simulink model "sampleModel161"  (R2021b)
settings: Solver=VariableStepAuto  StartTime=0.0  StopTime=10.0  RelTol=1e-3
undefined symbols (not defined in the file or in its folder): DiscIntNeverNeededParam
libraries: simulink x19, slpidlib x1
settings Model: Creator=user  LastModifiedBy=user

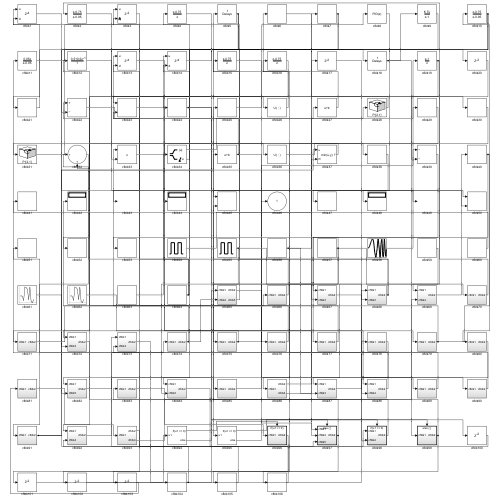
[thumbnail: Simulink's stored preview of the top-level diagram]
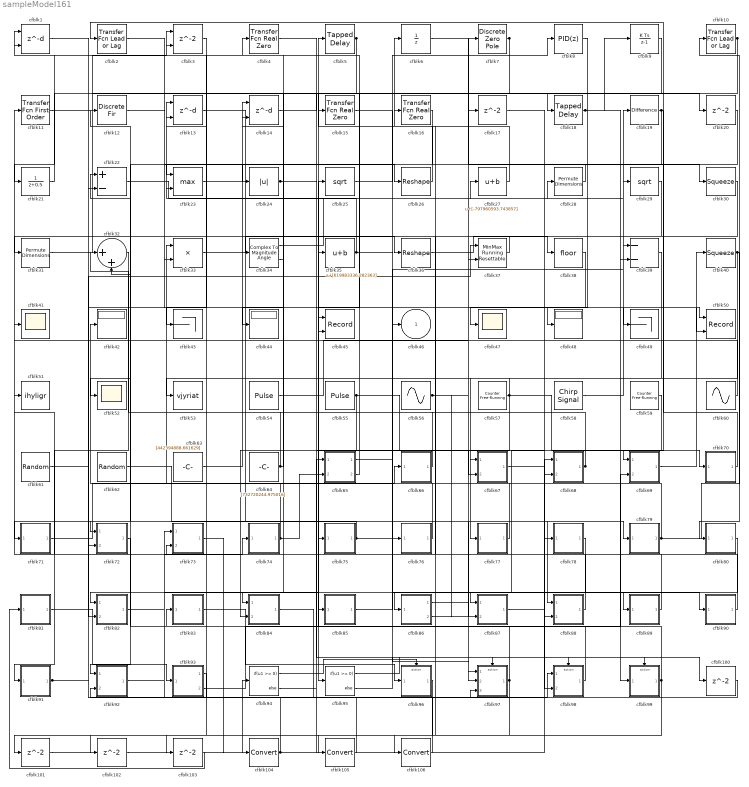
== system sampleModel161 ==
  cfblk1 : Delay  DelayLengthSource=Input port  SampleTime=1
      settings: InputPortMap=u0,p1
  cfblk10 : simulink/Discrete/Transfer Fcn Lead or Lag  PoleZ=0.95  ZeroZ=0.75  ICPrevOutput=0.0  ICPrevInput=0.0  DoSatur=off
      settings: SourceProductBaseCode=SL
  cfblk{17,20,100..103} (6 alike) : Delay  SampleTime=1
  cfblk104 : DataTypeConversion
  cfblk105 : DataTypeConversion
  cfblk106 : DataTypeConversion
  cfblk11 : simulink/Discrete/Transfer Fcn First Order  PoleZ=0.95  ICPrevOutput=0.0  DoSatur=off
  cfblk12 : DiscreteFir  SampleTime=1
  cfblk13 : Delay  DelayLengthSource=Input port  SampleTime=1
      settings: InputPortMap=u0,p1
  cfblk14 : Delay  DelayLengthSource=Input port  SampleTime=1
      settings: InputPortMap=u0,p1
  cfblk15 : simulink/Discrete/Transfer Fcn Real Zero  ZeroZ=0.75  ICPrevInput=0.0  DoSatur=off
      settings: SourceProductBaseCode=SL
  cfblk16 : simulink/Discrete/Transfer Fcn Real Zero  ZeroZ=0.75  ICPrevInput=0.0  DoSatur=off
      settings: SourceProductBaseCode=SL
  cfblk18 : simulink/Discrete/Tapped Delay  vinit=0.0  samptime=-1  NumDelays=1  DelayOrder=Oldest  includeCurrent=off
  cfblk19 : simulink/Discrete/Difference  ICPrevInput=0.0  OutMin=[]  OutMax=[]  OutDataTypeStr=Inherit: Inherit via back propagation  OutDataType=fixdt(1, 16)  OutScaling=2^-10  DoSatur=off
  cfblk2 : simulink/Discrete/Transfer Fcn Lead or Lag  PoleZ=0.95  ZeroZ=0.75  ICPrevOutput=0.0  ICPrevInput=0.0  DoSatur=off
      settings: SourceProductBaseCode=SL
  cfblk21 : DiscreteTransferFcn  SampleTime=1
  cfblk22 : Sum  Inputs=+-
  cfblk23 : MinMax  Function=max  Inputs=2
  cfblk24 : Abs
  cfblk25 : Sqrt  SaturateOnIntegerOverflow=on
  cfblk26 : Reshape
  cfblk27 : Bias  Bias=[-797960593.743857]
  cfblk28 : PermuteDimensions
  cfblk29 : Sqrt  SaturateOnIntegerOverflow=on
  cfblk3 : Delay  ShowEnablePort=on  SampleTime=1
      settings: InputPortMap=u0,e6
  cfblk30 : Squeeze
  cfblk31 : PermuteDimensions
  cfblk32 : Sum  Inputs=|++
  cfblk33 : Product  Inputs=**
  cfblk34 : ComplexToMagnitudeAngle
  cfblk35 : Bias  Bias=[619983336.282363]
  cfblk36 : Reshape
  cfblk37 : simulink/Math Operations/MinMax Running Resettable  Function=min  vinit=0.0
  cfblk38 : Rounding
  cfblk39 : Sum  Inputs=--
  cfblk4 : simulink/Discrete/Transfer Fcn Real Zero  ZeroZ=0.75  ICPrevInput=0.0  DoSatur=off
      settings: SourceProductBaseCode=SL
  cfblk40 : Squeeze
  cfblk41 : Scope
  cfblk42 : Display
  cfblk43 : Terminator
  cfblk44 : Display
  cfblk45 : Record  FileSettingsInternal="{\"entries\":[{\"content\":{\"excelSettings\":{\"content\":{},\"type\":\"Streamout.ExcelSettings\"}},\"type\":\"Streamout.FileSettingStorage\",\"uuid\":\"aea9327c-655b-48bd-a78c-8c98bb394b7e\"}],\"packageUris\":[\"http://schema.mathworks.com/mf0/streamout_blocks/R2020a\"],\"version\":\"1.0\"}"  Layout=[1 1]  SignalsInternal="{\"entries\":[{\"content\":{\"signals\":[{\"content\":{\"blockPath\":[\"sampleModel161/cfblk45\"],\"channel\":[],\"dimensions\":[1],\"domain\":\"sampleModel161/cfblk45\",\"lineColor\":\"#a2142f\",\"plots\":[1],\"port\":1,\"sid\":[\"\"],\"signalID\":6094,\"signalName\":\"cfblk10\"},\"type\":\"RecordBlkView.Signal\",\"uuid\":\"d1a2102a-b012-4f36-9f7c-29bbfcbaf4f0\"},{\"content\":{\"blockPath\":[\"sampleModel161/cfblk45\"],\"channel\":[],\"dimensions\":[1],\"domain\":\"sampleModel161/cfblk45\",\"lineColor\":\"#139fff\",\"plots\":[1],\"port\":2,\"sid\":[\"\"],\"signalID\":6100,\"signalName\":\"cfblk68\"},\"type\":\"RecordBlkView.Signal\",\"uuid\":\"a18f6999-1e72-4cfb-8c53-260dab68c9ad\"}]},\"type\":\"RecordBlkView.InputSignals\",\"uuid\":\"b3fefcdd-efa0-42cd-ad0d-6efafa40c42e\"}],\"packageUris\":[\"http://schema.mathworks.com/mf0/streamout_blocks/R2020a\"],\"version\":\"1.0\"}"  VisualizationBindings="{\"xyplotplugin\":{\"info\":[{\"series\":[{\"bindingParametersList\":[{\"parameter\":\"X-Axis\",\"signalID\":6094,\"signalName\":\"cfblk10\"},{\"parameter\":\"Y-Axis\",\"signalID\":6100,\"signalName\":\"cfblk68\"}],\"seriesID\":50617}],\"subplotID\":1}]}}"  CompatibilityTag=XY
  cfblk47 : Scope
  cfblk48 : Display
  cfblk49 : Terminator
  cfblk5 : simulink/Discrete/Tapped Delay  vinit=0.0  samptime=-1  NumDelays=1  DelayOrder=Oldest  includeCurrent=off
  cfblk50 : Record  FileSettingsInternal="{\"entries\":[{\"content\":{\"excelSettings\":{\"content\":{},\"type\":\"Streamout.ExcelSettings\"}},\"type\":\"Streamout.FileSettingStorage\",\"uuid\":\"217729ac-a3b3-492b-8907-d0a7c10fa8f5\"}],\"packageUris\":[\"http://schema.mathworks.com/mf0/streamout_blocks/R2020a\"],\"version\":\"1.0\"}"  Layout=[1 1]  SignalsInternal="{\"entries\":[{\"content\":{\"signals\":[{\"content\":{\"blockPath\":[\"sampleModel161/cfblk50\"],\"channel\":[],\"dimensions\":[1],\"domain\":\"sampleModel161/cfblk50\",\"lineColor\":\"#a2142f\",\"plots\":[1],\"port\":1,\"sid\":[\"\"],\"signalID\":6104,\"signalName\":\"cfblk1\"},\"type\":\"RecordBlkView.Signal\",\"uuid\":\"d3e4b2a0-8b34-436e-97c2-dbcffd0622e8\"},{\"content\":{\"blockPath\":[\"sampleModel161/cfblk50\"],\"channel\":[],\"dimensions\":[1],\"domain\":\"sampleModel161/cfblk50\",\"lineColor\":\"#139fff\",\"plots\":[1],\"port\":2,\"sid\":[\"\"],\"signalID\":6108,\"signalName\":\"cfblk24\"},\"type\":\"RecordBlkView.Signal\",\"uuid\":\"f67a0d4e-4bac-4f1a-913f-2d5f37e423fc\"}]},\"type\":\"RecordBlkView.InputSignals\",\"uuid\":\"93948432-514c-4838-bd97-bd51c83fe33b\"}],\"packageUris\":[\"http://schema.mathworks.com/mf0/streamout_blocks/R2020a\"],\"version\":\"1.0\"}"  VisualizationBindings="{\"xyplotplugin\":{\"info\":[{\"series\":[{\"bindingParametersList\":[{\"parameter\":\"X-Axis\",\"signalID\":6104,\"signalName\":\"cfblk1\"},{\"parameter\":\"Y-Axis\",\"signalID\":6108,\"signalName\":\"cfblk24\"}],\"seriesID\":40753}],\"subplotID\":1}]}}"  CompatibilityTag=XY
  cfblk51 : ToWorkspace  VariableName=ihyligr  SaveFormat=Timeseries  SampleTime=-1
  cfblk52 : Scope
  cfblk53 : ToWorkspace  VariableName=vjyriat  SaveFormat=Timeseries  SampleTime=-1
  cfblk54 : DiscretePulseGenerator  PulseType=Time based  Amplitude=[902121356.280096]  Period=[53508103.241336]  PulseWidth=5  PhaseDelay=[9.000000]
  cfblk55 : DiscretePulseGenerator  PulseType=Time based  Amplitude=[269668819.301766]  Period=[58775580.792966]  PulseWidth=5  PhaseDelay=[5.000000]
  cfblk56 : Sin  Amplitude=[-709093241.756912]  Bias=[-149963615.888180]  SampleTime=0
  cfblk57 : simulink/Sources/Counter Free-Running  NumBits=[39.000000]  tsamp=-1
  cfblk58 : simulink/Sources/Chirp Signal  f1=[-797958734.286313]  T=[-186043220.453092]  f2=[610396473.545557]
  cfblk59 : simulink/Sources/Counter Free-Running  NumBits=[41.000000]  tsamp=-1
  cfblk6 : UnitDelay  HasFrameUpgradeWarning=on
  cfblk60 : Sin  Amplitude=[665714232.719712]  Bias=[-960226317.803523]  SampleTime=0
  cfblk61 : RandomNumber  Mean=[-57210.883663]  Variance=[49850.840022]  Seed=[517220069.000000]  SampleTime=0.1
  cfblk62 : RandomNumber  Mean=[62654.103054]  Variance=[86318.692322]  Seed=[86968229.000000]  SampleTime=0.1
  cfblk63 : Constant  Value=[442394888.661629]  SampleTime=1
  cfblk64 : Constant  Value=[732720244.975016]  SampleTime=1
  cfblk65 : Subsystem
  cfblk66 : Subsystem
  cfblk67 : Subsystem
  cfblk68 : Subsystem
  cfblk69 : Subsystem
  cfblk7 : DiscreteZeroPole  Poles=[0 0.5]  Gain=1
  cfblk70 : Subsystem
  cfblk71 : Subsystem
  cfblk72 : Subsystem
  cfblk73 : Subsystem
  cfblk74 : Subsystem
  cfblk75 : Subsystem
  cfblk76 : Subsystem
  cfblk77 : Subsystem
  cfblk78 : Subsystem
  cfblk79 : Subsystem
  cfblk8 : slpidlib/PID Controller  Controller=PID  Form=Parallel  TimeDomain=Discrete-time  UseExternalTs=off  SampleTime=1  IntegratorMethod=Forward Euler  FilterMethod=Forward Euler  ControllerParametersSource=internal  P=1  I=1  D=0  UseFilter=on  N=100  TunerSelectOption=Transfer Function Based (PID Tuner App)  InitialConditionSource=internal  InitialConditionForIntegrator=0  InitialConditionForFilter=0  DifferentiatorICPrevScaledInput=0  ExternalReset=none  TrackingMode=off  Kt=1  LimitOutput=off  SatLimitsSource=internal  UpperSaturationLimit=inf  LowerSaturationLimit=-inf  LinearizeAsGain=off  AntiWindupMode=none  Kb=1  POutMin=[]  POutMax=[]  IOutMin=[]  IOutMax=[]  DOutMin=[]  DOutMax=[]  NOutMin=[]  NOutMax=[]  SumOutMin=[]  SumOutMax=[]  SaturationOutMin=[]  SaturationOutMax=[]  PParamMin=[]  PParamMax=[]  IParamMin=[]  IParamMax=[]  DParamMin=[]  DParamMax=[]  NParamMin=[]  NParamMax=[]  KbParamMin=[]  KbParamMax=[]  KtParamMin=[]  KtParamMax=[]  KbOutMin=[]  KbOutMax=[]  KtOutMin=[]  KtOutMax=[]  IntegratorOutMin=[]  IntegratorOutMax=[]  FilterOutMin=[]  FilterOutMax=[]  SumI1OutMin=[]  SumI1OutMax=[]  SumI2OutMin=[]  SumI2OutMax=[]  SumI3OutMin=[]  SumI3OutMax=[]  SumI4OutMin=[]  SumI4OutMax=[]  SumDOutMin=[]  SumDOutMax=[]  DifferentiatorOutMin=[]  DifferentiatorOutMax=[]  FilterDiffOutCoefMin=[]  FilterDiffOutCoefMax=[]  ReciprocalOutMin=[]  ReciprocalOutMax=[]  SumDenOutMin=[]  SumDenOutMax=[]  SumNumOutMin=[]  SumNumOutMax=[]  DivideOutMin=[]  DivideOutMax=[]  UdiffTsProdOutMin=[]  UdiffTsProdOutMax=[]  NTsProdOutMin=[]  NTsProdOutMax=[]  UintegralTsProdOutMin=[]  UintegralTsProdOutMax=[]  UngainTsProdOutMin=[]  UngainTsProdOutMax=[]  IntegratorContinuousStateAttributes=''  IntegratorStateMustResolveToSignalObject=off  IntegratorRTWStateStorageClass=Auto  FilterContinuousStateAttributes=''  FilterStateMustResolveToSignalObject=off  FilterRTWStateStorageClass=Auto  ParallelPVariant=InternalParameters  IdealPVariant=Disabled  IVariant=InternalParameters  DVariant=InternalParameters  IntegratorVariant=Discrete  SatVariant=Disabled  AWVariant=Passthrough  PCopyVariant=Disabled  TRVariant=Disabled  FdbkBlocksVariant=Forward  IdealPFdbkVariant=Disabled  SatFdbkVariant=Disabled  DerivativeFilterVariant=ForwardEulerFilter  NVariant=InternalParameters  NCopyVariant=Disabled  FilterICVariant=InternalICsFilter  IntegratorICVariant=InternalICs  ExternalResetVariant=Disabled  TRSumVariant=Passthrough  SumFdbkVariant=Disabled  SumVariant=Sum_PID  TsampFilterVariant=InternalTs  TsampNgainVariant=Passthrough  TsampIntegralVariant=Passthrough  ExternalSaturationOutDataTypeStr=Inherit: Same as second input
  cfblk80 : Subsystem
  cfblk81 : Subsystem
  cfblk82 : Subsystem
  cfblk83 : Subsystem
  cfblk84 : Subsystem
  cfblk85 : Subsystem
  cfblk86 : Subsystem
  cfblk87 : Subsystem
  cfblk88 : Subsystem
  cfblk89 : Subsystem
  cfblk9 : DiscreteIntegrator  ICPrevOutput=DiscIntNeverNeededParam  ICPrevScaledInput=DiscIntNeverNeededParam
  cfblk90 : Subsystem
  cfblk91 : Subsystem
  cfblk92 : Subsystem
  cfblk93 : Subsystem
  cfblk94 : If  IfExpression=u1 >= 0  SampleTime=1
  cfblk95 : If  IfExpression=u1 >= 0  SampleTime=1
  cfblk96 : Subsystem  TreatAsAtomicUnit=on
  cfblk97 : Subsystem  TreatAsAtomicUnit=on
  cfblk98 : Subsystem  TreatAsAtomicUnit=on
  cfblk99 : Subsystem  TreatAsAtomicUnit=on
  cfblk46 : Outport
  wires:
  cfblk74/1(cfblk2) -> cfblk42/1, cfblk65/2(cfblk4)
  cfblk35/1 -> cfblk13/1, cfblk97/2(cfblk4)
  cfblk39/1 -> cfblk77/1(cfblk1)
  cfblk57/1 -> cfblk70/1(cfblk1), cfblk53/1, cfblk84/2(cfblk3), cfblk106/1
  cfblk89/1(cfblk2) -> cfblk11/1
  cfblk7/1 -> cfblk95/1, cfblk72/2(cfblk3)
  cfblk70/1(cfblk2) -> cfblk2/1
  cfblk84/1(cfblk2) -> cfblk98/1(cfblk1)
  cfblk28/1 -> cfblk23/1
  cfblk38/1 -> cfblk47/1
  cfblk71/1(cfblk2) -> cfblk66/1(cfblk1)
  cfblk58/1 -> cfblk19/1
  cfblk83/1(cfblk2) -> cfblk96/1(cfblk1)
  cfblk9/1 -> cfblk21/1
  cfblk75/1(cfblk2) -> cfblk71/1(cfblk1), cfblk39/1
  cfblk31/1 -> cfblk3/1
  cfblk81/1(cfblk2) -> cfblk93/1(cfblk1)
  cfblk80/1(cfblk2) -> cfblk82/1(cfblk1)
  cfblk86/1(cfblk2) -> cfblk7/1
  cfblk11/1 -> cfblk18/1
  cfblk22/1 -> cfblk27/1
  cfblk62/1 -> cfblk88/1(cfblk1)
  cfblk65/1(cfblk2) -> cfblk90/1(cfblk1)
  cfblk34/1 -> cfblk29/1
  cfblk90/1(cfblk2) -> cfblk51/1
  cfblk77/1(cfblk2) -> cfblk13/2
  cfblk26/1 -> cfblk5/1
  cfblk87/1(cfblk2) -> cfblk78/1(cfblk1)
  cfblk18/1 -> cfblk99/1(cfblk1), cfblk9/1
  cfblk15/1 -> cfblk76/1(cfblk1)
  cfblk8/1 -> cfblk48/1
  cfblk78/1(cfblk2) -> cfblk98/2(cfblk4)
  cfblk60/1 -> cfblk41/1
  cfblk72/1(cfblk2) -> cfblk92/1(cfblk1)
  cfblk6/1 -> cfblk30/1
  cfblk54/1 -> cfblk17/1
  cfblk73/1(cfblk2) -> cfblk104/1
  cfblk65/2(cfblk5) -> cfblk4/1
  cfblk99/1(cfblk2) -> cfblk25/1, cfblk105/1
  cfblk59/1 -> cfblk87/1(cfblk1)
  cfblk79/1(cfblk2) -> cfblk10/1, cfblk12/1
  cfblk66/1(cfblk2) -> cfblk15/1
  cfblk97/1(cfblk2) -> cfblk22/1, cfblk102/1
  cfblk30/1 -> cfblk72/1(cfblk1)
  cfblk92/1(cfblk2) -> cfblk74/1(cfblk1)
  cfblk2/1 -> cfblk26/1
  cfblk27/1 -> cfblk6/1
  cfblk20/1 -> cfblk52/1
  cfblk29/1 -> cfblk86/1(cfblk1)
  cfblk98/1(cfblk2) -> cfblk83/1(cfblk1)
  cfblk88/1(cfblk2) -> cfblk16/1
  cfblk10/1 -> cfblk84/1(cfblk1), cfblk33/2, cfblk45/1
  cfblk21/1 -> cfblk1/1
  cfblk36/1 -> cfblk38/1
  cfblk55/1 -> cfblk75/1(cfblk1), cfblk67/2(cfblk3)
  cfblk24/1 -> cfblk68/2(cfblk3), cfblk50/2
  cfblk13/1 -> cfblk79/1(cfblk1)
  cfblk17/1 -> cfblk88/2(cfblk4)
  cfblk61/1 -> cfblk82/2(cfblk5)
  cfblk33/1 -> cfblk36/1
  cfblk23/1 -> cfblk97/1(cfblk1)
  cfblk34/2 -> cfblk1/2
  cfblk40/1 -> cfblk80/1(cfblk1), cfblk67/1(cfblk1)
  cfblk1/1 -> cfblk50/1
  cfblk19/1 -> cfblk69/1(cfblk1), cfblk39/2
  cfblk68/1(cfblk2) -> cfblk32/1, cfblk45/2
  cfblk12/1 -> cfblk49/1
  cfblk67/1(cfblk2) -> cfblk89/1(cfblk1)
  cfblk86/2(cfblk4) -> cfblk28/1
  cfblk63/1 -> cfblk14/1
  cfblk69/1(cfblk2) -> cfblk40/1
  cfblk82/1(cfblk2) -> cfblk85/1(cfblk1)
  cfblk16/1 -> cfblk32/2
  cfblk25/1 -> cfblk8/1
  cfblk91/1(cfblk2) -> cfblk37/1, cfblk35/1, cfblk97/3(cfblk5)
  cfblk32/1 -> cfblk91/1(cfblk1)
  cfblk93/2(cfblk4) -> cfblk69/2(cfblk4)
  cfblk76/1(cfblk2) -> cfblk33/1
  cfblk3/1 -> cfblk43/1
  cfblk56/1 -> cfblk37/2, cfblk87/2(cfblk3)
  cfblk85/1(cfblk2) -> cfblk46/1
  cfblk5/1 -> cfblk22/2, cfblk44/1, cfblk24/1
  cfblk14/1 -> cfblk20/1
  cfblk64/1 -> cfblk34/1, cfblk14/2, cfblk23/2
  cfblk37/1 -> cfblk31/1
  cfblk94/1 -> cfblk96/Action
  cfblk94/2 -> cfblk97/Action
  cfblk95/1 -> cfblk98/Action
  cfblk95/2 -> cfblk99/Action
  cfblk4/1 -> cfblk100/1
  cfblk100/1 -> cfblk92/2(cfblk4)
  cfblk96/1(cfblk2) -> cfblk101/1
  cfblk101/1 -> cfblk68/1(cfblk1)
  cfblk102/1 -> cfblk94/1
  cfblk93/1(cfblk2) -> cfblk103/1
  cfblk103/1 -> cfblk81/1(cfblk1)
  cfblk104/1 -> cfblk65/1(cfblk1), cfblk3/2
  cfblk105/1 -> cfblk73/1(cfblk1)
  cfblk106/1 -> cfblk73/2(cfblk4)

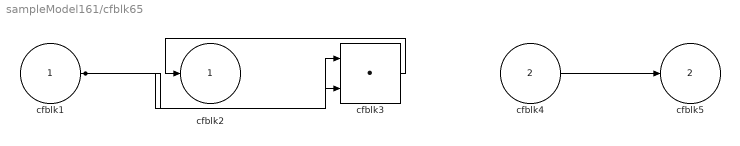
== system sampleModel161/cfblk65 ==
  cfblk1 : Inport
  cfblk4 : Inport  Port=2
  cfblk3 : DotProduct  InputSameDT=on  OutDataTypeStr=Inherit: Inherit via internal rule
  cfblk2 : Outport
  cfblk5 : Outport  Port=2
  wires:
  cfblk3/1 -> cfblk2/1
  cfblk4/1 -> cfblk5/1
  cfblk1/1 -> cfblk3/1, cfblk3/2

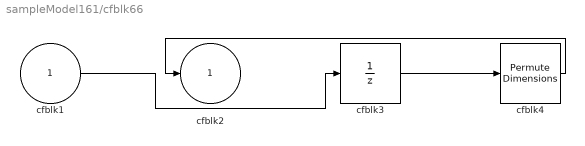
== system sampleModel161/cfblk66 ==
  cfblk1 : Inport
  cfblk3 : UnitDelay  HasFrameUpgradeWarning=on
  cfblk4 : PermuteDimensions
  cfblk2 : Outport
  wires:
  cfblk3/1 -> cfblk4/1
  cfblk4/1 -> cfblk2/1
  cfblk1/1 -> cfblk3/1

== system sampleModel161/cfblk67 ==
  cfblk1 : Inport
  cfblk3 : Inport  Port=2
  cfblk2 : Outport
  wires:
  cfblk3/1 -> cfblk2/1

== system sampleModel161/cfblk68 ==
  cfblk1 : Inport
  cfblk3 : Inport  Port=2
  cfblk2 : Outport
  wires:
  cfblk3/1 -> cfblk2/1

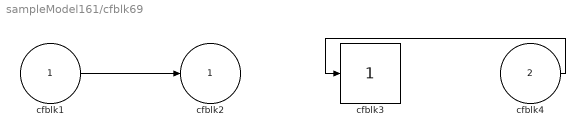
== system sampleModel161/cfblk69 ==
  cfblk1 : Inport
  cfblk4 : Inport  Port=2
  cfblk3 : simulink/Math Operations/Slider Gain  gain=1  low=0  high=2
  cfblk2 : Outport
  wires:
  cfblk1/1 -> cfblk2/1
  cfblk4/1 -> cfblk3/1

== system sampleModel161/cfblk70 ==
  cfblk1 : Inport
  cfblk3 : UnitDelay  HasFrameUpgradeWarning=on
  cfblk2 : Outport
  wires:
  cfblk1/1 -> cfblk3/1
  cfblk3/1 -> cfblk2/1

== system sampleModel161/cfblk71 ==
  cfblk1 : Inport
  cfblk3 : Gain  Gain=[-781035660.055184]
  cfblk2 : Outport
  wires:
  cfblk1/1 -> cfblk2/1, cfblk3/1

== system sampleModel161/cfblk72 ==
  cfblk1 : Inport
  cfblk3 : Inport  Port=2
  cfblk2 : Outport
  wires:
  cfblk1/1 -> cfblk2/1

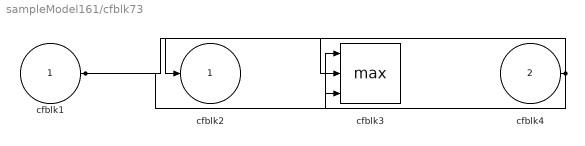
== system sampleModel161/cfblk73 ==
  cfblk1 : Inport
  cfblk4 : Inport  Port=2
  cfblk3 : MinMax  Function=max  Inputs=3
  cfblk2 : Outport
  wires:
  cfblk4/1 -> cfblk2/1, cfblk3/3
  cfblk1/1 -> cfblk3/1, cfblk3/2

== system sampleModel161/cfblk74 ==
  cfblk1 : Inport
  cfblk3 : simulink/Discrete/Transfer Fcn Lead or Lag  PoleZ=0.95  ZeroZ=0.75  ICPrevOutput=0.0  ICPrevInput=0.0  DoSatur=off
      settings: SourceProductBaseCode=SL
  cfblk2 : Outport
  wires:
  cfblk1/1 -> cfblk3/1
  cfblk3/1 -> cfblk2/1

== system sampleModel161/cfblk75 ==
  cfblk1 : Inport
  cfblk3 : simulink/Discrete/Difference  ICPrevInput=0.0  OutMin=[]  OutMax=[]  OutDataTypeStr=Inherit: Inherit via back propagation  OutDataType=fixdt(1, 16)  OutScaling=2^-10  DoSatur=off
  cfblk4 : Sqrt  SaturateOnIntegerOverflow=on
  cfblk2 : Outport
  wires:
  cfblk3/1 -> cfblk4/1
  cfblk4/1 -> cfblk2/1
  cfblk1/1 -> cfblk3/1

== system sampleModel161/cfblk76 ==
  cfblk1 : Inport
  cfblk3 : Math  Operator=log  SaturateOnIntegerOverflow=on
  cfblk2 : Outport
  wires:
  cfblk1/1 -> cfblk2/1, cfblk3/1

== system sampleModel161/cfblk77 ==
  cfblk1 : Inport
  cfblk3 : DiscreteFilter  SampleTime=1
  cfblk2 : Outport
  wires:
  cfblk1/1 -> cfblk3/1
  cfblk3/1 -> cfblk2/1

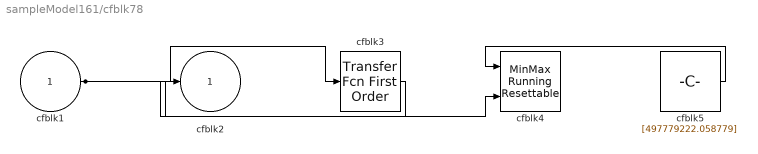
== system sampleModel161/cfblk78 ==
  cfblk1 : Inport
  cfblk3 : simulink/Discrete/Transfer Fcn First Order  PoleZ=0.95  ICPrevOutput=0.0  DoSatur=off
  cfblk4 : simulink/Math Operations/MinMax Running Resettable  Function=min  vinit=0.0
  cfblk5 : Constant  Value=[497779222.058779]  SampleTime=1
  cfblk2 : Outport
  wires:
  cfblk1/1 -> cfblk3/1, cfblk4/2
  cfblk5/1 -> cfblk4/1
  cfblk3/1 -> cfblk2/1

== system sampleModel161/cfblk79 ==
  cfblk1 : Inport
  cfblk3 : DiscreteFir  SampleTime=1
  cfblk4 : Constant  Value=[635149472.487827]  SampleTime=1
  cfblk2 : Outport
  wires:
  cfblk4/1 -> cfblk2/1
  cfblk1/1 -> cfblk3/1

== system sampleModel161/cfblk80 ==
  cfblk1 : Inport
  cfblk3 : Sum  Inputs=--
  cfblk4 : Constant  Value=[-282751784.938534]  SampleTime=1
  cfblk2 : Outport
  wires:
  cfblk1/1 -> cfblk2/1, cfblk3/2
  cfblk4/1 -> cfblk3/1

== system sampleModel161/cfblk81 ==
  cfblk1 : Inport
  cfblk3 : Delay  SampleTime=1
  cfblk4 : Abs
  cfblk2 : Outport
  wires:
  cfblk3/1 -> cfblk4/1
  cfblk1/1 -> cfblk3/1
  cfblk4/1 -> cfblk2/1

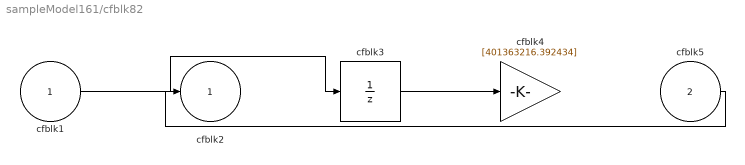
== system sampleModel161/cfblk82 ==
  cfblk1 : Inport
  cfblk5 : Inport  Port=2
  cfblk3 : UnitDelay  HasFrameUpgradeWarning=on
  cfblk4 : Gain  Gain=[401363216.392434]
  cfblk2 : Outport
  wires:
  cfblk1/1 -> cfblk3/1
  cfblk5/1 -> cfblk2/1
  cfblk3/1 -> cfblk4/1

== system sampleModel161/cfblk83 ==
  cfblk1 : Inport
  cfblk3 : PermuteDimensions
  cfblk2 : Outport
  wires:
  cfblk1/1 -> cfblk3/1
  cfblk3/1 -> cfblk2/1

== system sampleModel161/cfblk84 ==
  cfblk1 : Inport
  cfblk3 : Inport  Port=2
  cfblk2 : Outport
  wires:
  cfblk3/1 -> cfblk2/1

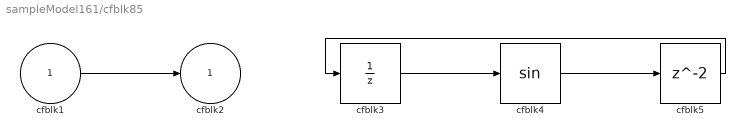
== system sampleModel161/cfblk85 ==
  cfblk1 : Inport
  cfblk3 : UnitDelay  HasFrameUpgradeWarning=on
  cfblk4 : Trigonometry
  cfblk5 : Delay  SampleTime=1
  cfblk2 : Outport
  wires:
  cfblk1/1 -> cfblk2/1
  cfblk3/1 -> cfblk4/1
  cfblk4/1 -> cfblk5/1
  cfblk5/1 -> cfblk3/1

== system sampleModel161/cfblk86 ==
  cfblk1 : Inport
  cfblk3 : DiscreteIntegrator  ICPrevOutput=DiscIntNeverNeededParam  ICPrevScaledInput=DiscIntNeverNeededParam
  cfblk2 : Outport
  cfblk4 : Outport  Port=2
  wires:
  cfblk1/1 -> cfblk4/1, cfblk3/1
  cfblk3/1 -> cfblk2/1

== system sampleModel161/cfblk87 ==
  cfblk1 : Inport
  cfblk3 : Inport  Port=2
  cfblk2 : Outport
  wires:
  cfblk3/1 -> cfblk2/1

== system sampleModel161/cfblk88 ==
  cfblk1 : Inport
  cfblk4 : Inport  Port=2
  cfblk3 : Signum
  cfblk2 : Outport
  wires:
  cfblk4/1 -> cfblk3/1
  cfblk3/1 -> cfblk2/1

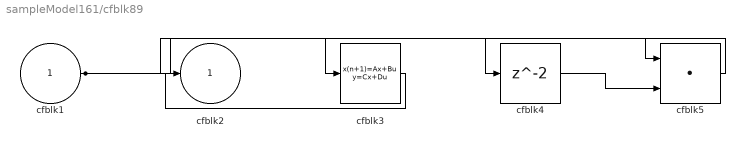
== system sampleModel161/cfblk89 ==
  cfblk1 : Inport
  cfblk3 : DiscreteStateSpace
  cfblk4 : Delay  SampleTime=1
  cfblk5 : DotProduct  InputSameDT=on  OutDataTypeStr=Inherit: Inherit via internal rule
  cfblk2 : Outport
  wires:
  cfblk1/1 -> cfblk5/1, cfblk4/1
  cfblk3/1 -> cfblk2/1
  cfblk5/1 -> cfblk3/1
  cfblk4/1 -> cfblk5/2

== system sampleModel161/cfblk90 ==
  cfblk1 : Inport
  cfblk3 : Reshape
  cfblk2 : Outport
  wires:
  cfblk1/1 -> cfblk3/1
  cfblk3/1 -> cfblk2/1

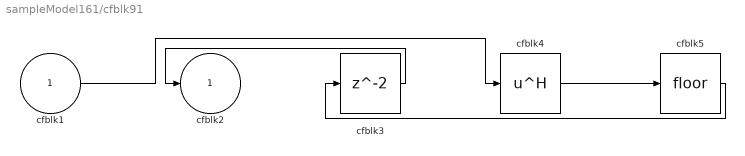
== system sampleModel161/cfblk91 ==
  cfblk1 : Inport
  cfblk3 : Delay  SampleTime=1
  cfblk4 : Math  Operator=hermitian  SaturateOnIntegerOverflow=on
  cfblk5 : Rounding
  cfblk2 : Outport
  wires:
  cfblk3/1 -> cfblk2/1
  cfblk5/1 -> cfblk3/1
  cfblk1/1 -> cfblk4/1
  cfblk4/1 -> cfblk5/1

== system sampleModel161/cfblk92 ==
  cfblk1 : Inport
  cfblk4 : Inport  Port=2
  cfblk3 : Constant  Value=[-141331307.999933]  SampleTime=1
  cfblk2 : Outport
  wires:
  cfblk3/1 -> cfblk2/1

== system sampleModel161/cfblk93 ==
  cfblk1 : Inport
  cfblk3 : DotProduct  InputSameDT=on  OutDataTypeStr=Inherit: Inherit via internal rule
  cfblk2 : Outport
  cfblk4 : Outport  Port=2
  wires:
  cfblk3/1 -> cfblk2/1
  cfblk1/1 -> cfblk3/1, cfblk4/1, cfblk3/2

== system sampleModel161/cfblk96 ==
  cfblk1 : Inport
  Action Port : ActionPort  ActionPortLabel=if(u1 >= 0)
  cfblk3 : Sqrt  SaturateOnIntegerOverflow=on
  cfblk2 : Outport
  wires:
  cfblk1/1 -> cfblk2/1, cfblk3/1

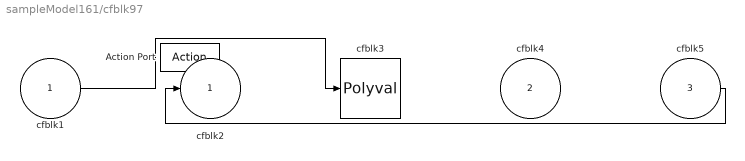
== system sampleModel161/cfblk97 ==
  cfblk1 : Inport
  cfblk4 : Inport  Port=2
  cfblk5 : Inport  Port=3
  Action Port : ActionPort  ActionPortLabel=else
  cfblk3 : Polyval  Coefs=[ +2.081618890e-019, -1.441693666e-014, +4.719686976e-010, -8.536869453e-006, +1.621573104e-001, -8.087801117e+001 ]
  cfblk2 : Outport
  wires:
  cfblk5/1 -> cfblk2/1
  cfblk1/1 -> cfblk3/1

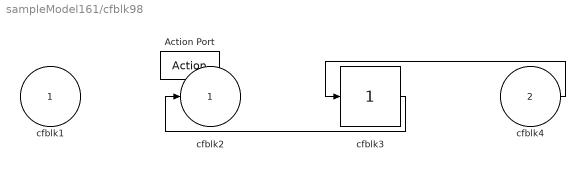
== system sampleModel161/cfblk98 ==
  cfblk1 : Inport
  cfblk4 : Inport  Port=2
  Action Port : ActionPort  ActionPortLabel=if(u1 >= 0)
  cfblk3 : simulink/Math Operations/Slider Gain  gain=1  low=0  high=2
  cfblk2 : Outport
  wires:
  cfblk3/1 -> cfblk2/1
  cfblk4/1 -> cfblk3/1

== system sampleModel161/cfblk99 ==
  cfblk1 : Inport
  Action Port : ActionPort  ActionPortLabel=else
  cfblk3 : DotProduct  InputSameDT=on  OutDataTypeStr=Inherit: Inherit via internal rule
  cfblk2 : Outport
  wires:
  cfblk1/1 -> cfblk3/1, cfblk3/2
  cfblk3/1 -> cfblk2/1
